simulink model "closed_loop3"  (R2012b)
settings: Solver=ode3  StartTime=0.0  StopTime=t_total+60  FixedStep=0.001  RelTol=1e-3
values from neighbouring files (symbols this model uses):
  a = D/(8*(t1^2)*(n^2))    [Craneparameters.m]    (also in Craneparameters2.m = 0.428041999052; Craneparameters3.m = 0.428041999052; Craneparameters4.m = 0.5; Craneparameters5.m = 0.428041999052)
  A1 = 1/(1+P)    [Craneparameters4.m]
  A2 = P/(1+P)    [Craneparameters4.m]
  D = 100    [Craneparameters.m]    (also in Craneparameters2.m; Craneparameters3.m = 129.5952; Craneparameters4.m = 120; Craneparameters5.m = 108.49)
  g = 9.81    [Craneparameters.m]    (also in Craneparameters2.m; Craneparameters3.m; Craneparameters4.m; Craneparameters5.m)
  K = 2/w    [Craneparameters4.m]    (also in Craneparameters5.m; Prototype_parameters.m; Slidingmode.m)
  l = 40    [Craneparameters.m]    (also in Craneparameters2.m; Craneparameters3.m; Craneparameters4.m; Craneparameters5.m)
  M = 26*10^3    (= 26000)    [Craneparameters.m]    (also in Craneparameters2.m; Craneparameters3.m; Craneparameters4.m; Craneparameters5.m)
  m = 67.3*10^3    (= 67300)    [Craneparameters.m]    (also in Craneparameters2.m; Craneparameters3.m; Craneparameters4.m; Craneparameters5.m)
  T1 = n*T    [Craneparameters.m]    (also in Craneparameters2.m; Craneparameters3.m; Craneparameters4.m = t1; Craneparameters5.m)
  t1 = T/4    [Craneparameters.m]    (also in Craneparameters2.m; Craneparameters3.m; Craneparameters4.m = round(100*Vmax/a)/100; Craneparameters5.m)
  T2 = n*T+t2    [Craneparameters.m]    (also in Craneparameters2.m; Craneparameters3.m = (n+1)*T; Craneparameters4.m = t1+t2; Craneparameters5.m = (n+1)*T)
  t_total = 2*n*T + t2    [Craneparameters.m]    (also in Craneparameters2.m = t_total2; Craneparameters3.m = 2*(n+1)*T + t2; Craneparameters4.m = T2+t1; Craneparameters5.m = 2*(n+1)*T + t2)
  Vmax = 3    [Craneparameters.m]    (also in Craneparameters2.m; Craneparameters3.m; Craneparameters4.m = 2.8; Craneparameters5.m)
libraries: simulink x2
settings Model: Creator=mchusr  LastModifiedBy=mchusr

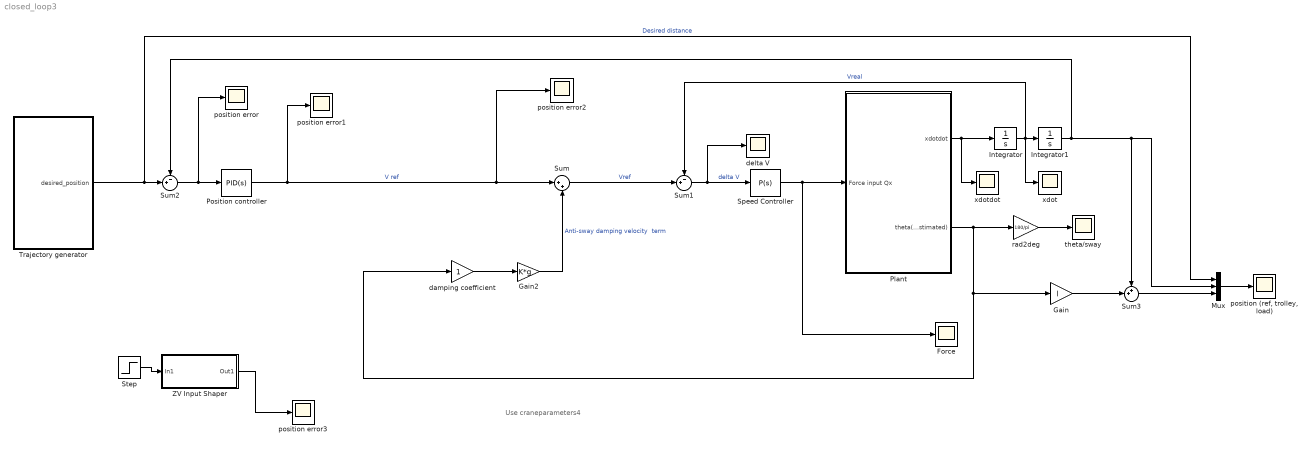
== system closed_loop3 ==
  note: Use craneparameters4
  Force : Scope
      settings: TimeRange=105  YMin=-600000  YMax=100000  SaveName=xdotdot1
  Gain : Gain  Gain=l
  Gain2 : Gain  Gain=K*g
  Integrator : Integrator
  Integrator1 : Integrator
  Mux : Mux  Inputs=3
  Plant : Subsystem
  Position controller : simulink/Continuous/PID Controller  Controller=PID  TimeDomain=Continuous-time  SampleTime=1  IntegratorMethod=Forward Euler  FilterMethod=Forward Euler  Form=Parallel  P=3  I=0.08  D=8  N=100  InitialConditionSource=internal  InitialConditionForIntegrator=0  InitialConditionForFilter=0  ExternalReset=none  LimitOutput=off  UpperSaturationLimit=inf  LowerSaturationLimit=-inf  LinearizeAsGain=on  AntiWindupMode=none  Kb=1  TrackingMode=off  Kt=1  PParamMin=[]  PParamMax=[]  IParamMin=[]  IParamMax=[]  DParamMin=[]  DParamMax=[]  NParamMin=[]  NParamMax=[]  KbParamMin=[]  KbParamMax=[]  KtParamMin=[]  KtParamMax=[]  POutMin=[]  POutMax=[]  IOutMin=[]  IOutMax=[]  DOutMin=[]  DOutMax=[]  NOutMin=[]  NOutMax=[]  KbOutMin=[]  KbOutMax=[]  KtOutMin=[]  KtOutMax=[]  IntegratorOutMin=[]  IntegratorOutMax=[]  FilterOutMin=[]  FilterOutMax=[]  SumOutMin=[]  SumOutMax=[]  SumI1OutMin=[]  SumI1OutMax=[]  SumI2OutMin=[]  SumI2OutMax=[]  SumI3OutMin=[]  SumI3OutMax=[]  SumDOutMin=[]  SumDOutMax=[]  SaturationOutMin=[]  SaturationOutMax=[]  IntegratorContinuousStateAttributes=''  IntegratorStateMustResolveToSignalObject=off  IntegratorRTWStateStorageClass=Auto  FilterContinuousStateAttributes=''  FilterStateMustResolveToSignalObject=off  FilterRTWStateStorageClass=Auto
  Speed Controller : simulink/Continuous/PID Controller  Controller=P  TimeDomain=Continuous-time  SampleTime=1  IntegratorMethod=Forward Euler  FilterMethod=Forward Euler  Form=Parallel  P=(M+m)  I=10*(M+m)  D=(M+m)  N=100  InitialConditionSource=internal  InitialConditionForIntegrator=0  InitialConditionForFilter=0  ExternalReset=none  LimitOutput=off  UpperSaturationLimit=inf  LowerSaturationLimit=-inf  LinearizeAsGain=on  AntiWindupMode=none  Kb=1  TrackingMode=off  Kt=1  PParamMin=[]  PParamMax=[]  IParamMin=[]  IParamMax=[]  DParamMin=[]  DParamMax=[]  NParamMin=[]  NParamMax=[]  KbParamMin=[]  KbParamMax=[]  KtParamMin=[]  KtParamMax=[]  POutMin=[]  POutMax=[]  IOutMin=[]  IOutMax=[]  DOutMin=[]  DOutMax=[]  NOutMin=[]  NOutMax=[]  KbOutMin=[]  KbOutMax=[]  KtOutMin=[]  KtOutMax=[]  IntegratorOutMin=[]  IntegratorOutMax=[]  FilterOutMin=[]  FilterOutMax=[]  SumOutMin=[]  SumOutMax=[]  SumI1OutMin=[]  SumI1OutMax=[]  SumI2OutMin=[]  SumI2OutMax=[]  SumI3OutMin=[]  SumI3OutMax=[]  SumDOutMin=[]  SumDOutMax=[]  SaturationOutMin=[]  SaturationOutMax=[]  IntegratorContinuousStateAttributes=''  IntegratorStateMustResolveToSignalObject=off  IntegratorRTWStateStorageClass=Auto  FilterContinuousStateAttributes=''  FilterStateMustResolveToSignalObject=off  FilterRTWStateStorageClass=Auto
  Step : Step  SampleTime=0
  Sum : Sum  Inputs=|++
  Sum1 : Sum  Inputs=-+|
  Sum2 : Sum  Inputs=-+|
  Sum3 : Sum  Inputs=++|
  Trajectory generator : Subsystem
  ZV Input Shaper : Subsystem
  damping coefficient : Gain
  delta V : Scope
      settings: TimeRange=105  YMin=-7.5e-08  YMax=7.5e-08  SaveName=xdotdot3
  "position (ref, trolley, load)" : Scope
      settings: TimeRange=105  SaveName=position2
  position error{,1..3} (4 alike) : Scope
      position error settings: TimeRange=105  YMin=-7.5e-08  YMax=7.5e-08  SaveName=xdotdot2
      position error1 settings: TimeRange=105  YMin=-0.25  YMax=0.25  SaveName=xdotdot4
      position error2 settings: TimeRange=105  YMin=-0.5  YMax=2.25  SaveName=xdotdot5
      position error3 settings: TimeRange=105  YMin=-0.25  YMax=0.25  SaveName=xdotdot9
  rad2deg : Gain  Gain=180/pi
  theta/sway : Scope
      settings: SaveName=sway2
  xdot : Scope
      settings: TimeRange=64.833  YMin=5.55112e-17  YMax=1.9  SaveName=velocity
  xdotdot : Scope
      settings: TimeRange=105  YMin=-7.5e-08  YMax=7.5e-08  SaveName=xdotdot
  wires:
  Plant/1(xdotdot) -> Integrator/1, xdotdot/1
  Integrator/1 -> Sum1/1, xdot/1, Integrator1/1  "Vreal"
  Integrator1/1 -> Mux/2, Sum3/1, Sum2/1
  Plant/2(theta(estimated)) -> rad2deg/1, Gain/1, damping coefficient/1
  Speed Controller/1 -> Plant/1(Force input Qx), Force/1
  Position controller/1 -> position error2/1, Sum/1, position error1/1  "V ref"
  Gain2/1 -> Sum/2  "Anti-sway damping velocity  term"
  damping coefficient/1 -> Gain2/1
  Sum/1 -> Sum1/2  "Vref"
  Sum1/1 -> delta V/1, Speed Controller/1  "delta V"
  Sum2/1 -> Position controller/1, position error/1
  Trajectory generator/1(desired_position) -> Mux/1, Sum2/2  "Desired distance"
  rad2deg/1 -> theta/sway/1
  Gain/1 -> Sum3/2
  Sum3/1 -> Mux/3
  Mux/1 -> "position (ref, trolley, load)"/1
  ZV Input Shaper/1(Out1) -> position error3/1
  Step/1 -> ZV Input Shaper/1(In1)

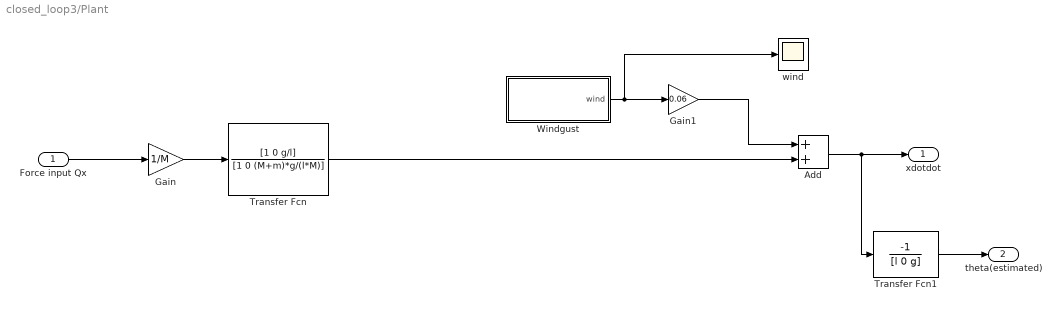
== system closed_loop3/Plant ==
  Force input Qx : Inport
  Add : Sum
  Gain : Gain  Gain=1/M
  Gain1 : Gain  Gain=0.06
  Transfer Fcn : TransferFcn  Numerator=[1 0 g/l]  Denominator=[1 0 (M+m)*g/(l*M)]
  Transfer Fcn1 : TransferFcn  Numerator=[-1]  Denominator=[l 0 g]
  Windgust : Subsystem
  wind : Scope
      settings: SaveName=wind
  xdotdot : Outport
  theta(estimated) : Outport  Port=2
  wires:
  Force input Qx/1 -> Gain/1
  Gain/1 -> Transfer Fcn/1
  Transfer Fcn/1 -> Add/2
  Transfer Fcn1/1 -> theta(estimated)/1
  Windgust/1(wind) -> wind/1, Gain1/1
  Add/1 -> Transfer Fcn1/1, xdotdot/1
  Gain1/1 -> Add/1

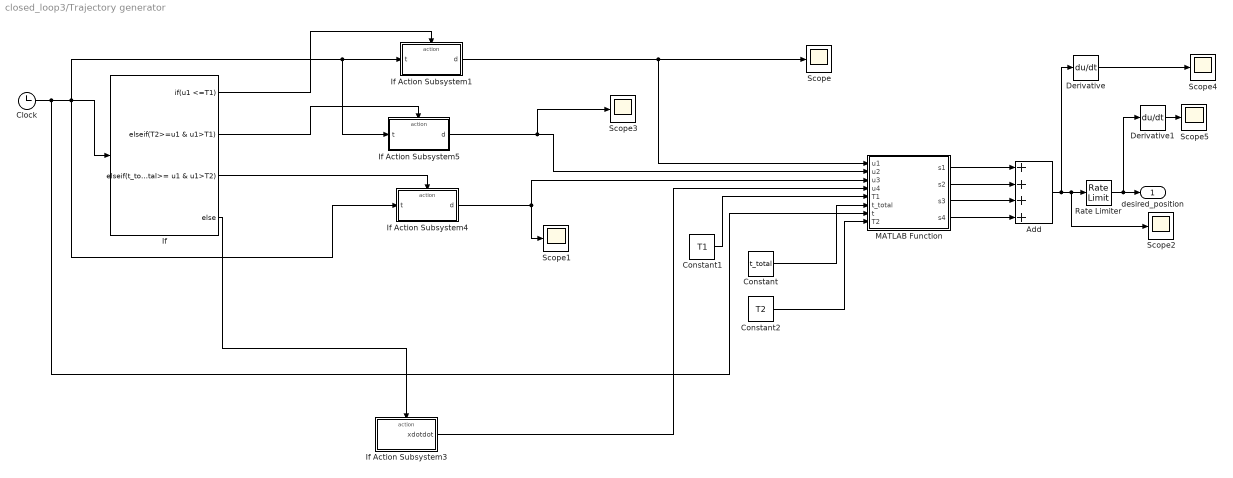
== system closed_loop3/Trajectory generator ==
  Add : Sum  Inputs=++++
  Clock : Clock
  Constant : Constant  Value=t_total
  Constant1 : Constant  Value=T1
  Constant2 : Constant  Value=T2
  Derivative : Derivative
  Derivative1 : Derivative
  If : If  IfExpression=u1 <=T1  ElseIfExpressions=T2>=u1 & u1>T1, t_total>= u1 & u1>T2  ZeroCross=off
  If Action Subsystem1 : Subsystem  TreatAsAtomicUnit=on
  If Action Subsystem3 : Subsystem  TreatAsAtomicUnit=on
  If Action Subsystem4 : Subsystem  TreatAsAtomicUnit=on
  If Action Subsystem5 : Subsystem  TreatAsAtomicUnit=on
  MATLAB Function : MATLAB Function  TreatAsAtomicUnit=on
  Rate Limiter : RateLimiter  RisingSlewLimit=Vmax  FallingSlewLimit=-Vmax  SampleTimeMode=inherited
  Scope{,1..5} (6 alike) : Scope
      Scope settings: SaveName=ScopeData4
      Scope1 settings: SaveName=ScopeData5
      Scope2 settings: YMin=10  YMax=100  SaveName=ref
      Scope4 settings: YMin=10  YMax=100  SaveName=ref1
      Scope5 settings: YMin=10  YMax=100  SaveName=ref2
  desired_position : Outport
  wires:
  If/1 -> If Action Subsystem1/Action
  If/2 -> If Action Subsystem5/Action
  If/3 -> If Action Subsystem4/Action
  Clock/1 -> MATLAB Function/7(t), If Action Subsystem4/1(t), If Action Subsystem5/1(t), If Action Subsystem1/1(t), If/1
  Add/1 -> Derivative/1, Scope2/1, Rate Limiter/1
  If Action Subsystem5/1(d) -> Scope3/1, MATLAB Function/2(u2)
  If Action Subsystem4/1(d) -> MATLAB Function/3(u3), Scope1/1
  If Action Subsystem3/1(xdotdot) -> MATLAB Function/4(u4)
  If/4 -> If Action Subsystem3/Action
  If Action Subsystem1/1(d) -> MATLAB Function/1(u1), Scope/1
  MATLAB Function/1(s1) -> Add/1
  MATLAB Function/2(s2) -> Add/2
  MATLAB Function/3(s3) -> Add/3
  MATLAB Function/4(s4) -> Add/4
  Constant1/1 -> MATLAB Function/5(T1)
  Constant/1 -> MATLAB Function/6(t_total)
  Constant2/1 -> MATLAB Function/8(T2)
  Derivative/1 -> Scope4/1
  Rate Limiter/1 -> Derivative1/1, desired_position/1
  Derivative1/1 -> Scope5/1

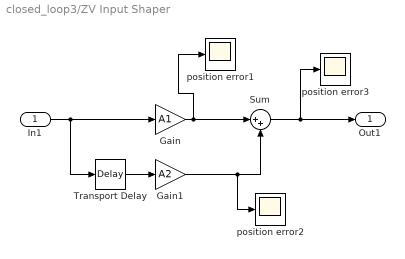
== system closed_loop3/ZV Input Shaper ==
  In1 : Inport
  Gain : Gain  Gain=A1
  Gain1 : Gain  Gain=A2
  Sum : Sum  Inputs=|++
  Transport Delay : TransportDelay  DelayTime=t  BufferSize=7268
  position error1 : Scope
      settings: TimeRange=105  YMin=-0.5  YMax=2.25  SaveName=xdotdot7
  position error2 : Scope
      settings: TimeRange=105  YMin=-0.5  YMax=2.25  SaveName=xdotdot6
  position error3 : Scope
      settings: TimeRange=105  YMin=-0.5  YMax=2.25  SaveName=xdotdot8
  Out1 : Outport
  wires:
  In1/1 -> Transport Delay/1, Gain/1
  Transport Delay/1 -> Gain1/1
  Gain/1 -> position error1/1, Sum/1
  Gain1/1 -> position error2/1, Sum/2
  Sum/1 -> position error3/1, Out1/1

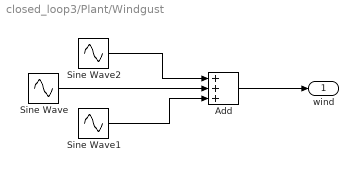
== system closed_loop3/Plant/Windgust ==
  Add : Sum  Inputs=+++
  Sine Wave : Sin  Amplitude=5  Frequency=0.2  SampleTime=0
  Sine Wave1 : Sin  Amplitude=3  Frequency=0.3  Phase=1  SampleTime=0
  Sine Wave2 : Sin  Phase=2.04  SampleTime=0
  wind : Outport
  wires:
  Sine Wave2/1 -> Add/1
  Sine Wave/1 -> Add/2
  Sine Wave1/1 -> Add/3
  Add/1 -> wind/1

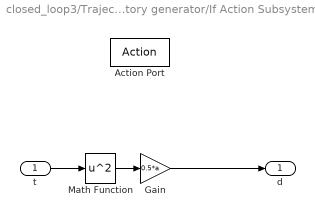
== system closed_loop3/Trajectory generator/If Action Subsystem1 ==
  t : Inport
  Action Port : ActionPort  ActionType=then
  Gain : Gain  Gain=0.5*a
  Math Function : Math  Operator=square  SaturateOnIntegerOverflow=on
  d : Outport
  wires:
  Gain/1 -> d/1
  t/1 -> Math Function/1
  Math Function/1 -> Gain/1

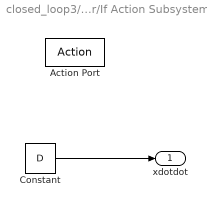
== system closed_loop3/Trajectory generator/If Action Subsystem3 ==
  Action Port : ActionPort  ActionType=else
  Constant : Constant  Value=D
  xdotdot : Outport
  wires:
  Constant/1 -> xdotdot/1

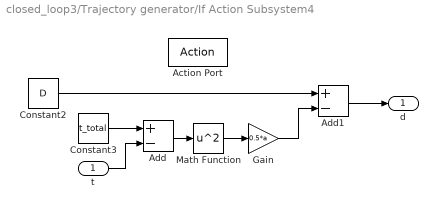
== system closed_loop3/Trajectory generator/If Action Subsystem4 ==
  t : Inport
  Action Port : ActionPort  ActionType=elseif
  Add : Sum  Inputs=+-
  Add1 : Sum  Inputs=+-
  Constant2 : Constant  Value=D
  Constant3 : Constant  Value=t_total
  Gain : Gain  Gain=0.5*a
  Math Function : Math  Operator=square  SaturateOnIntegerOverflow=on
  d : Outport
  wires:
  Math Function/1 -> Gain/1
  Constant3/1 -> Add/1
  t/1 -> Add/2
  Add/1 -> Math Function/1
  Constant2/1 -> Add1/1
  Gain/1 -> Add1/2
  Add1/1 -> d/1

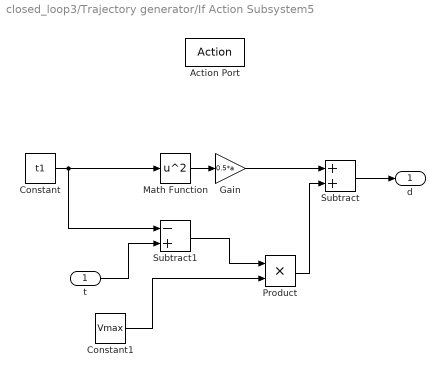
== system closed_loop3/Trajectory generator/If Action Subsystem5 ==
  t : Inport
  Action Port : ActionPort  ActionType=elseif
  Constant : Constant  Value=t1
  Constant1 : Constant  Value=Vmax
  Gain : Gain  Gain=0.5*a
  Math Function : Math  Operator=square  SaturateOnIntegerOverflow=on
  Product : Product  RndMeth=Zero
  Subtract : Sum
  Subtract1 : Sum  Inputs=-+
  d : Outport
  wires:
  Constant/1 -> Math Function/1, Subtract1/1
  Math Function/1 -> Gain/1
  Gain/1 -> Subtract/1
  t/1 -> Subtract1/2
  Constant1/1 -> Product/2
  Product/1 -> Subtract/2
  Subtract/1 -> d/1
  Subtract1/1 -> Product/1

== matlab function closed_loop3/Trajectory generator/MATLAB Function ==
  data: u1 input; s1 output; u2 input; u3 input; u4 input; T1 input; t_total input; s2 output; s3 output; s4 output; t input; T2 input
function [s1, s2, s3, s4] = filter(u1, u2, u3, u4, T1, t_total, t, T2)

if t<=T1
    s1 = u1;
else
    s1=0;
end

if t>T2
    s2 = 0;
else
    s2=u2;
end



if t<=t_total
    s3 = u3;
else
    s3=0;
end

if t>t_total
    s4 = u4;
else
    s4=0;
end




end
